simulink model "CM4_ADC_IMU_All"  (R2020b)
settings: Solver=FixedStepDiscrete  StartTime=0.0  StopTime=inf  FixedStep=0.001  RelTol=1e-3  EnableMultiTasking=on
libraries: simulink x9, raspberrypiCommlib x2, embdlinuxlib x1
settings Model: ModifiedByFormat=The MathWorks Inc.  SimulationMode=external  EnablePacing=on  Creator=The MathWorks, Inc.  LastModifiedBy=The MathWorks Inc.
settings SolverCC: PositivePriorityOrder=on
settings DataIOCC: LimitDataPoints=on  SaveFormat=Array  ReturnWorkspaceOutputs=off
settings OptimizationCC: LifeSpan=1  MaxStackSize=64
settings DebuggingCC: UnderspecifiedInitializationDetection=Classic  MergeDetectMultiDrivingBlocksExec=none  SolverPrmCheckMsg=warning  AllowSymbolicDim=off  SFUnexpectedBacktrackingDiag=warning  SFNoUnconditionalDefaultTransitionDiag=warning  SFExecutionAtInitializationDiag=none  ArithmeticOperatorsInVariantConditions=warning
settings HardwareCC: ProdBitPerPointer=32  ProdBitPerSizeT=32  ProdBitPerPtrDiffT=32  ProdLargestAtomicInteger=Long  ProdLargestAtomicFloat=Double  ProdWordSize=32  ProdLongLongMode=on  ProdHWDeviceType=ARM Compatible->ARM Cortex
settings SFSimCC: SimUseLocalCustomCode=off  MATLABDynamicMemAlloc=off  CustomCodeUndefinedFunction=UseInterfaceOnly
settings RTWCC: Description=Embedded Coder  SystemTargetFile=ert.tlc  HardwareBoard=Raspberry Pi  TemplateMakefile=ert_default_tmf  RTWUseLocalCustomCode=off  Toolchain=GNU GCC Raspberry Pi
settings CodeAppCC: StateflowObjectComments=on
settings ERTTargetCC: MultiwordLength=2048  ERTCustomFileBanners=off  MatFileLogging=on  SupportContinuousTime=on  SupportNonInlinedSFcns=on  RemoveResetFunc=off  ModelStepFunctionPrototypeControlCompliant=off  ConvertIfToSwitch=off  SuppressUnreachableDefaultCases=off
settings ConfigComp: CovMetricSettings=dw  CovSaveCumulativeToWorkspaceVar=on  CovSaveSingleToWorkspaceVar=on  CovExternalEMLEnable=off  CovSFcnEnable=off

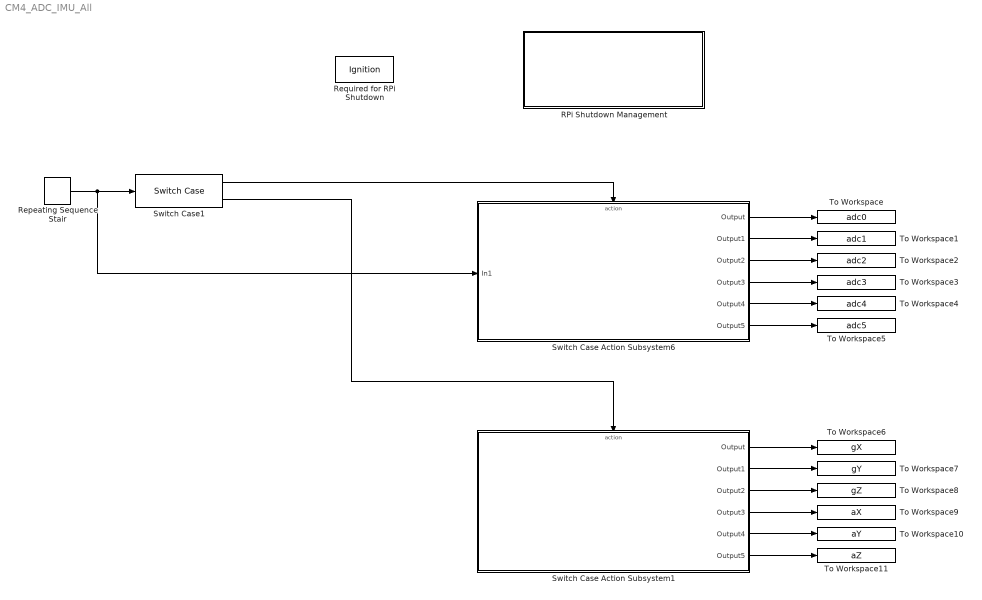
== system CM4_ADC_IMU_All ==
  RPi Shutdown Management : Subsystem
  Repeating Sequence Stair : simulink/Sources/Repeating Sequence Stair  OutValues=[0 1 2 3 4 5 6]'  tsamp=-1  OutMin=[]  OutMax=[]  OutDataTypeStr=double  OutputDataTypeScalingMode=double  OutDataType=fixdt(0,8)  ConRadixGroup=Best Precision: Vector-wise  OutScaling=2^-12
  Required for RPi Shutdown : DataStoreMemory  DataStoreName=Ignition  ReadBeforeWriteMsg=warning  WriteAfterWriteMsg=warning  WriteAfterReadMsg=warning  ShowAdditionalParam=off  OutDataTypeStr=uint8
  Switch Case Action Subsystem1 : Subsystem  TreatAsAtomicUnit=on
  Switch Case Action Subsystem6 : Subsystem  TreatAsAtomicUnit=on
  Switch Case1 : SwitchCase  CaseConditions={[0,1,2,3,4,5]}
  To Workspace : ToWorkspace  VariableName=adc0  SampleTime=-1
      settings: Save2DSignal=2-D array (concatenate along first dimension)
  To Workspace1 : ToWorkspace  VariableName=adc1  SampleTime=-1
      settings: Save2DSignal=2-D array (concatenate along first dimension)
  To Workspace10 : ToWorkspace  VariableName=aY  SampleTime=-1
      settings: Save2DSignal=2-D array (concatenate along first dimension)
  To Workspace11 : ToWorkspace  VariableName=aZ  SampleTime=-1
      settings: Save2DSignal=2-D array (concatenate along first dimension)
  To Workspace2 : ToWorkspace  VariableName=adc2  SampleTime=-1
      settings: Save2DSignal=2-D array (concatenate along first dimension)
  To Workspace3 : ToWorkspace  VariableName=adc3  SampleTime=-1
      settings: Save2DSignal=2-D array (concatenate along first dimension)
  To Workspace4 : ToWorkspace  VariableName=adc4  SampleTime=-1
      settings: Save2DSignal=2-D array (concatenate along first dimension)
  To Workspace5 : ToWorkspace  VariableName=adc5  SampleTime=-1
      settings: Save2DSignal=2-D array (concatenate along first dimension)
  To Workspace6 : ToWorkspace  VariableName=gX  SampleTime=-1
      settings: Save2DSignal=2-D array (concatenate along first dimension)
  To Workspace7 : ToWorkspace  VariableName=gY  SampleTime=-1
      settings: Save2DSignal=2-D array (concatenate along first dimension)
  To Workspace8 : ToWorkspace  VariableName=gZ  SampleTime=-1
      settings: Save2DSignal=2-D array (concatenate along first dimension)
  To Workspace9 : ToWorkspace  VariableName=aX  SampleTime=-1
      settings: Save2DSignal=2-D array (concatenate along first dimension)
  wires:
  Repeating Sequence Stair/1 -> Switch Case1/1, Switch Case Action Subsystem6/1(In1)
  Switch Case1/1 -> Switch Case Action Subsystem6/Action
  Switch Case1/2 -> Switch Case Action Subsystem1/Action
  Switch Case Action Subsystem6/1(Output) -> To Workspace/1
  Switch Case Action Subsystem6/2(Output1) -> To Workspace1/1
  Switch Case Action Subsystem6/3(Output2) -> To Workspace2/1
  Switch Case Action Subsystem6/4(Output3) -> To Workspace3/1
  Switch Case Action Subsystem6/5(Output4) -> To Workspace4/1
  Switch Case Action Subsystem6/6(Output5) -> To Workspace5/1
  Switch Case Action Subsystem1/1(Output) -> To Workspace6/1
  Switch Case Action Subsystem1/2(Output1) -> To Workspace7/1
  Switch Case Action Subsystem1/3(Output2) -> To Workspace8/1
  Switch Case Action Subsystem1/4(Output3) -> To Workspace9/1
  Switch Case Action Subsystem1/5(Output4) -> To Workspace10/1
  Switch Case Action Subsystem1/6(Output5) -> To Workspace11/1

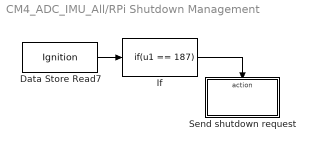
== system CM4_ADC_IMU_All/RPi Shutdown Management ==
  Data Store Read7 : DataStoreRead  DataStoreName=Ignition
  If : If  IfExpression=u1 == 187  ShowElse=off
  Send shutdown request : Subsystem  TreatAsAtomicUnit=on
  wires:
  If/1 -> Send shutdown request/Action
  Data Store Read7/1 -> If/1

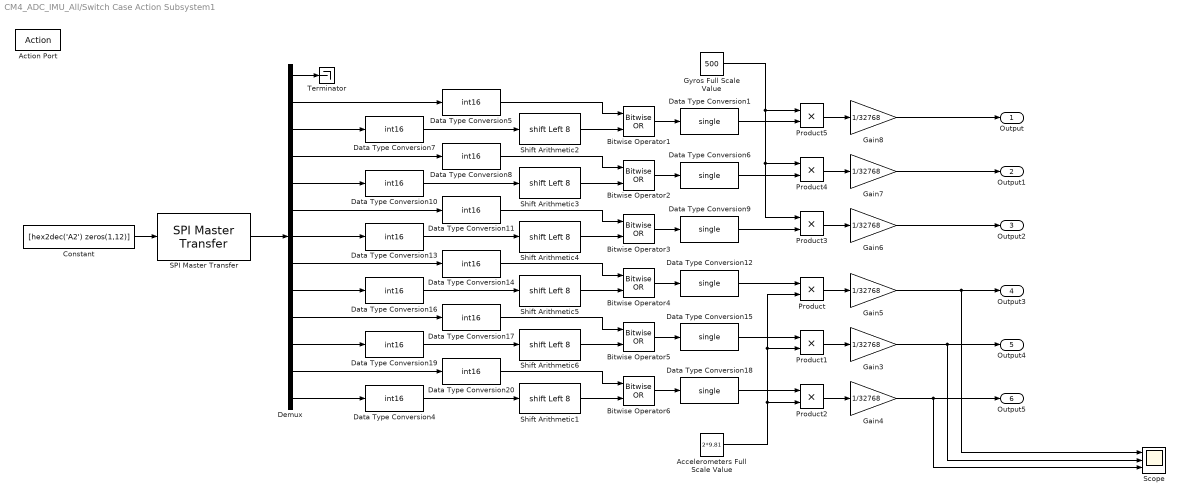
== system CM4_ADC_IMU_All/Switch Case Action Subsystem1 ==
  Action Port : ActionPort  ActionPortLabel=default:
  Accelerometers Full Scale Value : Constant  Value=2*9.81
  Bitwise Operator{1..6} (6 alike) : simulink/Logic and Bit Operations/Bitwise Operator  logicop=OR  UseBitMask=off  NumInputPorts=2  BitMask=bin2dec('11011001')  BitMaskRealWorld=Stored Integer
  Constant : Constant  Value=[hex2dec('A2') zeros(1,12)]  OutDataTypeStr=uint8
  Data Type Conversion{1,6,9,12,15,18} (6 alike) : DataTypeConversion  OutDataTypeStr=single
  Data Type Conversion{4..5,7..8,10..11,13..14,16..17,19..20} (12 alike) : DataTypeConversion  OutDataTypeStr=int16  ConvertRealWorld=Stored Integer (SI)
  Demux : Demux  Outputs=13
  Gain{3..8} (6 alike) : Gain  Gain=1/32768
  Gyros Full Scale Value : Constant  Value=500
  Product{,1..5} (6 alike) : Product
  SPI Master Transfer : raspberrypiCommlib/SPI Master Transfer  BoardProperty=Pi 4 Model B  SPIModule=SPI1  Mode=Master  BusSpeed=1000000  Pin=uint32(0)  FirstBitToTransfer=Most significant bit (MSB)  ClockMode=0  BlockFunction=Transfer  RegisterAddress=0  OutputDataType=int8  OutputDataLength=1  SSPin=CS2
      settings: SourceProductBaseCode=RASPPI
  Scope : Scope  NumInputPorts=3
  Shift Arithmetic{1..6} (6 alike) : ArithShift  BitShiftNumber=8  BitShiftDirection=Left
  Terminator : Terminator
  Output : Outport
  Output1 : Outport  Port=2
  Output2 : Outport  Port=3
  Output3 : Outport  Port=4
  Output4 : Outport  Port=5
  Output5 : Outport  Port=6
  wires:
  Demux/5 -> Data Type Conversion10/1
  Product5/1 -> Gain8/1
  Product1/1 -> Gain3/1
  Demux/11 -> Data Type Conversion19/1
  Data Type Conversion8/1 -> Bitwise Operator2/1
  Demux/10 -> Data Type Conversion17/1
  Demux/13 -> Data Type Conversion4/1
  Data Type Conversion16/1 -> Shift Arithmetic5/1
  Shift Arithmetic4/1 -> Bitwise Operator3/2
  Demux/6 -> Data Type Conversion11/1
  Constant/1 -> SPI Master Transfer/1
  Data Type Conversion6/1 -> Product4/2
  Product4/1 -> Gain7/1
  Gain3/1 -> Output4/1, Scope/2
  Shift Arithmetic3/1 -> Bitwise Operator2/2
  Data Type Conversion4/1 -> Shift Arithmetic1/1
  Product2/1 -> Gain4/1
  Data Type Conversion7/1 -> Shift Arithmetic2/1
  Demux/4 -> Data Type Conversion8/1
  Demux/7 -> Data Type Conversion13/1
  Data Type Conversion10/1 -> Shift Arithmetic3/1
  Data Type Conversion20/1 -> Bitwise Operator6/1
  Demux/9 -> Data Type Conversion16/1
  Demux/12 -> Data Type Conversion20/1
  Data Type Conversion5/1 -> Bitwise Operator1/1
  Data Type Conversion17/1 -> Bitwise Operator5/1
  Shift Arithmetic5/1 -> Bitwise Operator4/2
  Gyros Full Scale Value/1 -> Product5/1, Product4/1, Product3/1
  Shift Arithmetic1/1 -> Bitwise Operator6/2
  Demux/1 -> Terminator/1
  Bitwise Operator5/1 -> Data Type Conversion15/1
  Shift Arithmetic6/1 -> Bitwise Operator5/2
  Data Type Conversion11/1 -> Bitwise Operator3/1
  Data Type Conversion14/1 -> Bitwise Operator4/1
  SPI Master Transfer/1 -> Demux/1
  Bitwise Operator1/1 -> Data Type Conversion1/1
  Data Type Conversion19/1 -> Shift Arithmetic6/1
  Gain4/1 -> Output5/1, Scope/3
  Bitwise Operator4/1 -> Data Type Conversion12/1
  Demux/3 -> Data Type Conversion7/1
  Data Type Conversion9/1 -> Product3/2
  Shift Arithmetic2/1 -> Bitwise Operator1/2
  Gain8/1 -> Output/1
  Demux/2 -> Data Type Conversion5/1
  Gain7/1 -> Output1/1
  Data Type Conversion15/1 -> Product1/1
  Bitwise Operator6/1 -> Data Type Conversion18/1
  Data Type Conversion12/1 -> Product/1
  Product/1 -> Gain5/1
  Bitwise Operator3/1 -> Data Type Conversion9/1
  Data Type Conversion13/1 -> Shift Arithmetic4/1
  Data Type Conversion1/1 -> Product5/2
  Accelerometers Full Scale Value/1 -> Product2/2, Product1/2, Product/2
  Gain5/1 -> Output3/1, Scope/1
  Demux/8 -> Data Type Conversion14/1
  Data Type Conversion18/1 -> Product2/1
  Gain6/1 -> Output2/1
  Product3/1 -> Gain6/1
  Bitwise Operator2/1 -> Data Type Conversion6/1

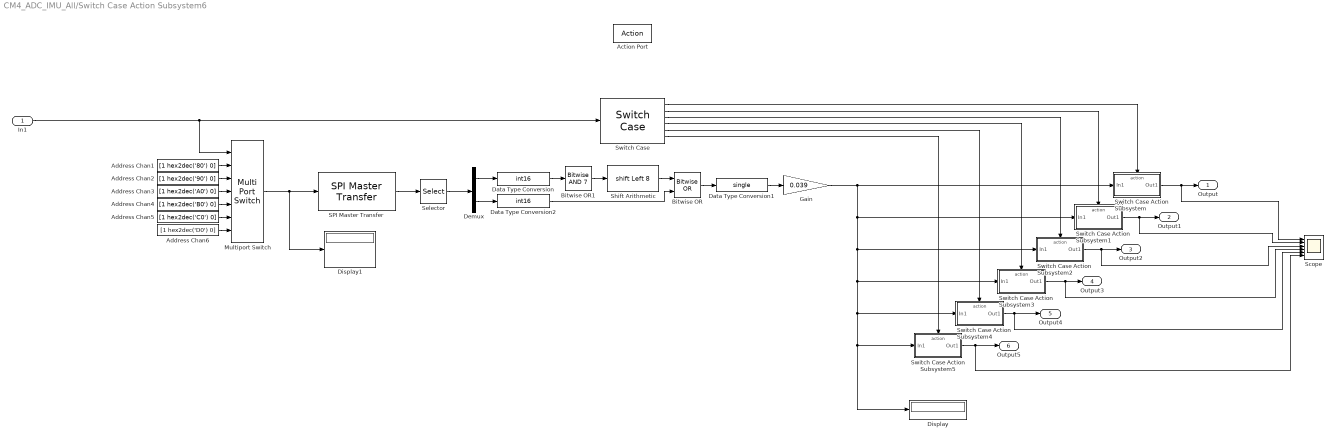
== system CM4_ADC_IMU_All/Switch Case Action Subsystem6 ==
  In1 : Inport
  Action Port : ActionPort  ActionPortLabel=case [ 0 1 2 3 4 5 ]:
  Address Chan1 : Constant  Value=[1 hex2dec('80') 0]  OutDataTypeStr=uint8
  Address Chan2 : Constant  Value=[1 hex2dec('90') 0]  OutDataTypeStr=uint8
  Address Chan3 : Constant  Value=[1 hex2dec('A0') 0]  OutDataTypeStr=uint8
  Address Chan4 : Constant  Value=[1 hex2dec('B0') 0]  OutDataTypeStr=uint8
  Address Chan5 : Constant  Value=[1 hex2dec('C0') 0]  OutDataTypeStr=uint8
  Address Chan6 : Constant  Value=[1 hex2dec('D0') 0]  OutDataTypeStr=uint8
  Bitwise OR : simulink/Logic and Bit Operations/Bitwise Operator  logicop=OR  UseBitMask=off  NumInputPorts=2  BitMask=bin2dec('11011001')  BitMaskRealWorld=Stored Integer
  Bitwise OR1 : simulink/Logic and Bit Operations/Bitwise Operator  logicop=AND  UseBitMask=on  BitMask=7  BitMaskRealWorld=Stored Integer
  Data Type Conversion : DataTypeConversion  OutDataTypeStr=int16
  Data Type Conversion1 : DataTypeConversion  OutDataTypeStr=single
  Data Type Conversion2 : DataTypeConversion  OutDataTypeStr=int16
  Demux : Demux  Outputs=2
  Display : Display
  Display1 : Display
  Gain : Gain  Gain=0.039
  Multiport Switch : MultiPortSwitch  DataPortOrder=Zero-based contiguous  Inputs=6  zeroidx=on  OutDataTypeStr=uint8
  SPI Master Transfer : raspberrypiCommlib/SPI Master Transfer  BoardProperty=Pi 4 Model B  SPIModule=SPI1  Mode=Master  BusSpeed=1000000  Pin=uint32(0)  FirstBitToTransfer=Most significant bit (MSB)  ClockMode=0  BlockFunction=Transfer  RegisterAddress=0  OutputDataType=int8  OutputDataLength=1  SSPin=CS1
      settings: SourceProductBaseCode=RASPPI
  Scope : Scope  NumInputPorts=6
  Selector : Selector  InputPortWidth=3  IndexOptions=Index vector (dialog)  Indices=[2 3]  OutputSizes=1
  Shift Arithmetic : ArithShift  BitShiftNumber=8  BitShiftDirection=Left
  Switch Case : SwitchCase  CaseConditions={0,1,2,3,4,5}  ShowDefaultCase=off
  Switch Case Action Subsystem : Subsystem  TreatAsAtomicUnit=on
  Switch Case Action Subsystem1 : Subsystem  TreatAsAtomicUnit=on
  Switch Case Action Subsystem2 : Subsystem  TreatAsAtomicUnit=on
  Switch Case Action Subsystem3 : Subsystem  TreatAsAtomicUnit=on
  Switch Case Action Subsystem4 : Subsystem  TreatAsAtomicUnit=on
  Switch Case Action Subsystem5 : Subsystem  TreatAsAtomicUnit=on
  Output : Outport
  Output1 : Outport  Port=2
  Output2 : Outport  Port=3
  Output3 : Outport  Port=4
  Output4 : Outport  Port=5
  Output5 : Outport  Port=6
  wires:
  Switch Case Action Subsystem1/1(Out1) -> Output1/1, Scope/2
  Switch Case/2 -> Switch Case Action Subsystem1/Action
  Address Chan1/1 -> Multiport Switch/2
  Switch Case Action Subsystem3/1(Out1) -> Output3/1, Scope/4
  Bitwise OR/1 -> Data Type Conversion1/1
  Switch Case/5 -> Switch Case Action Subsystem4/Action
  Demux/2 -> Data Type Conversion2/1
  Address Chan3/1 -> Multiport Switch/4
  In1/1 -> Multiport Switch/1, Switch Case/1
  Data Type Conversion1/1 -> Gain/1
  Data Type Conversion/1 -> Bitwise OR1/1
  Switch Case Action Subsystem2/1(Out1) -> Output2/1, Scope/3
  Switch Case Action Subsystem4/1(Out1) -> Output4/1, Scope/5
  Shift Arithmetic/1 -> Bitwise OR/1
  Address Chan6/1 -> Multiport Switch/7
  Multiport Switch/1 -> SPI Master Transfer/1, Display1/1
  Data Type Conversion2/1 -> Bitwise OR/2
  Bitwise OR1/1 -> Shift Arithmetic/1
  Switch Case/1 -> Switch Case Action Subsystem/Action
  SPI Master Transfer/1 -> Selector/1
  Switch Case Action Subsystem/1(Out1) -> Output/1, Scope/1
  Gain/1 -> Display/1, Switch Case Action Subsystem5/1(In1), Switch Case Action Subsystem4/1(In1), Switch Case Action Subsystem3/1(In1), Switch Case Action Subsystem2/1(In1), Switch Case Action Subsystem1/1(In1), Switch Case Action Subsystem/1(In1)
  Switch Case/6 -> Switch Case Action Subsystem5/Action
  Demux/1 -> Data Type Conversion/1
  Address Chan4/1 -> Multiport Switch/5
  Selector/1 -> Demux/1
  Address Chan5/1 -> Multiport Switch/6
  Address Chan2/1 -> Multiport Switch/3
  Switch Case/3 -> Switch Case Action Subsystem2/Action
  Switch Case/4 -> Switch Case Action Subsystem3/Action
  Switch Case Action Subsystem5/1(Out1) -> Output5/1, Scope/6

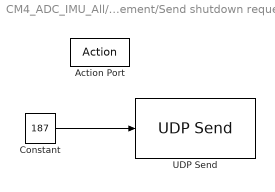
== system CM4_ADC_IMU_All/RPi Shutdown Management/Send shutdown request ==
  Action Port : ActionPort  ActionPortLabel=if(u1 == 187)
  Constant : Constant  Value=187  OutDataTypeStr=uint8
  UDP Send : embdlinuxlib/UDP Send  remoteURL='127.0.0.1'  remotePort=5005  localURL='255.255.255.255'  localPortSource=Automatically determine  localPort=-1  sampletime=-1  blockPlatform=Raspberry Pi  separateLengthPort=0
      settings: SourceProductBaseCode=SC_BEAGLEBONE_BLUE,NVIDIA,RASPPI
  wires:
  Constant/1 -> UDP Send/1

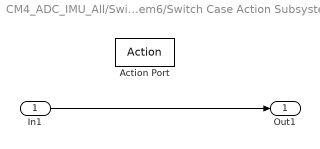
== system CM4_ADC_IMU_All/Switch Case Action Subsystem6/Switch Case Action Subsystem ==
  In1 : Inport
  Action Port : ActionPort  ActionPortLabel=case [ 0 ]:
  Out1 : Outport
  wires:
  In1/1 -> Out1/1

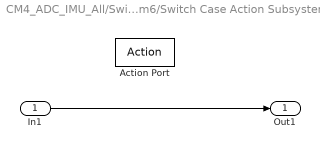
== system CM4_ADC_IMU_All/Switch Case Action Subsystem6/Switch Case Action Subsystem1 ==
  In1 : Inport
  Action Port : ActionPort  ActionPortLabel=case [ 1 ]:
  Out1 : Outport
  wires:
  In1/1 -> Out1/1

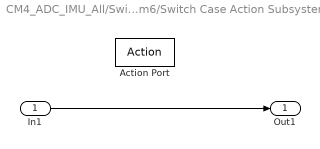
== system CM4_ADC_IMU_All/Switch Case Action Subsystem6/Switch Case Action Subsystem2 ==
  In1 : Inport
  Action Port : ActionPort  ActionPortLabel=case [ 2 ]:
  Out1 : Outport
  wires:
  In1/1 -> Out1/1

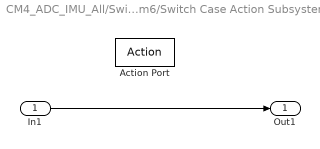
== system CM4_ADC_IMU_All/Switch Case Action Subsystem6/Switch Case Action Subsystem3 ==
  In1 : Inport
  Action Port : ActionPort  ActionPortLabel=case [ 3 ]:
  Out1 : Outport
  wires:
  In1/1 -> Out1/1

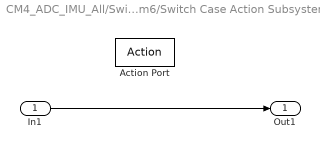
== system CM4_ADC_IMU_All/Switch Case Action Subsystem6/Switch Case Action Subsystem4 ==
  In1 : Inport
  Action Port : ActionPort  ActionPortLabel=case [ 4 ]:
  Out1 : Outport
  wires:
  In1/1 -> Out1/1

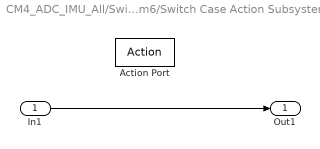
== system CM4_ADC_IMU_All/Switch Case Action Subsystem6/Switch Case Action Subsystem5 ==
  In1 : Inport
  Action Port : ActionPort  ActionPortLabel=case [ 5 ]:
  Out1 : Outport
  wires:
  In1/1 -> Out1/1
